simulink model "master_passivity_sys"  (R2015a)
settings: Solver=ode45  StartTime=0.0  StopTime=10  RelTol=1e-3
undefined symbols (not defined in the file): A, B, C, D, K
settings Model: Creator=enrico-giordano  LastModifiedBy=enrico-giordano

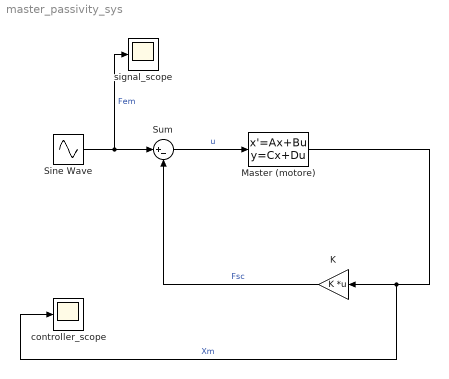
== system master_passivity_sys ==
  K : Gain  Gain=K  Multiplication=Matrix(K*u)
  Master (motore) : StateSpace  A=A  B=B  C=C  D=D  X0=0
  Sine Wave : Sin  Amplitude=10  SampleTime=0
  Sum : Sum  Inputs=|+-
  controller_scope : Scope
      settings: TimeRange=10  YMin=-0.6000000000000001  YMax=0.2  SaveName=ScopeData3
  signal_scope : Scope
      settings: TimeRange=10  YMin=-10  YMax=10
  wires:
  Sum/1 -> Master (motore)/1  "u"
  Sine Wave/1 -> signal_scope/1, Sum/1  "Fem"
  Master (motore)/1 -> controller_scope/1, K/1  "Xm"
  K/1 -> Sum/2  "Fsc"
